simulink library "LIB_AirVolumeProcessing"  (R2018b)
settings: Solver=VariableStepAuto  StartTime=0.0  StopTime=10.0  RelTol=1e-3
undefined symbols (not defined in the file or in its folder): eRespiratorStates, QAirDeadZoneThd
libraries: simulink x9
settings Model: Creator=BRAUL  LastModifiedBy=VITIE

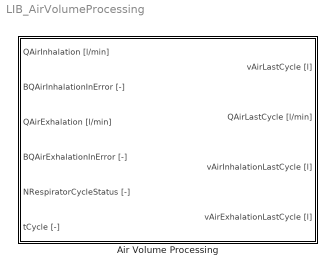
== system LIB_AirVolumeProcessing ==
  Air Volume Processing : Subsystem
      settings: AttributesFormatString=%<ReferenceBlock>

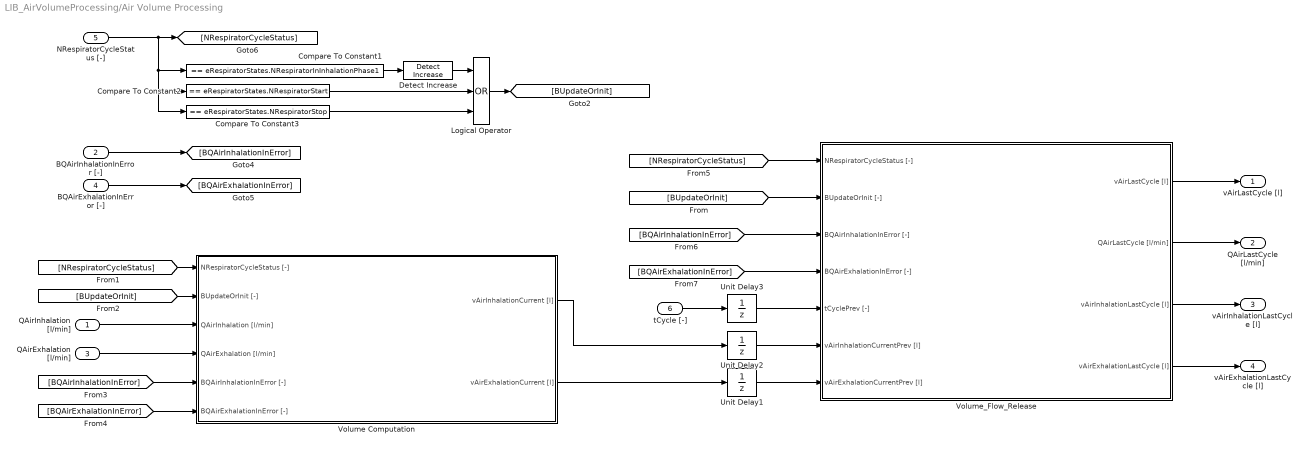
== system LIB_AirVolumeProcessing/Air Volume Processing ==
  QAirInhalation [l/min] : Inport
  BQAirInhalationInError [-] : Inport  Port=2
  QAirExhalation [l/min] : Inport  Port=3
  BQAirExhalationInError [-] : Inport  Port=4
  NRespiratorCycleStatus [-] : Inport  Port=5
  tCycle [-] : Inport  Port=6
  Compare To Constant1 : simulink/Logic and Bit Operations/Compare To Constant  relop===  const=eRespiratorStates.NRespiratorInInhalationPhase1  OutDataTypeStr=boolean
  Compare To Constant2 : simulink/Logic and Bit Operations/Compare To Constant  relop===  const=eRespiratorStates.NRespiratorStart  OutDataTypeStr=boolean
  Compare To Constant3 : simulink/Logic and Bit Operations/Compare To Constant  relop===  const=eRespiratorStates.NRespiratorStop  OutDataTypeStr=boolean
  Detect Increase : simulink/Logic and Bit Operations/Detect Increase  vinit=0.0  OutDataTypeStr=boolean
  Logical Operator : Logic  Operator=OR  Inputs=3  AllPortsSameDT=off  OutDataTypeStr=boolean
  Unit Delay1 : UnitDelay  SampleTime=-1
      settings: AttributesFormatString=%<InitialCondition>
  Unit Delay2 : UnitDelay  SampleTime=-1
      settings: AttributesFormatString=%<InitialCondition>
  Unit Delay3 : UnitDelay  SampleTime=-1
      settings: AttributesFormatString=%<InitialCondition>
  Volume Computation : Subsystem
  "Volume_Flow_Release " : Subsystem
  vAirLastCycle [l] : Outport
  QAirLastCycle [l/min] : Outport  Port=2
  vAirInhalationLastCycle [l] : Outport  Port=3
  vAirExhalationLastCycle [l] : Outport  Port=4
  wires:
  "Volume_Flow_Release "/3(vAirInhalationLastCycle [l]) -> vAirInhalationLastCycle [l]/1
  "Volume_Flow_Release "/4(vAirExhalationLastCycle [l]) -> vAirExhalationLastCycle [l]/1
  [BUpdateOrInit] -> "Volume_Flow_Release "/2(BUpdateOrInit [-])
  Compare To Constant3/1 -> Logical Operator/3
  Compare To Constant2/1 -> Logical Operator/2
  "Volume_Flow_Release "/1(vAirLastCycle [l]) -> vAirLastCycle [l]/1
  "Volume_Flow_Release "/2(QAirLastCycle [l/min]) -> QAirLastCycle [l/min]/1
  tCycle [-]/1 -> Unit Delay3/1
  Unit Delay3/1 -> "Volume_Flow_Release "/5(tCyclePrev [-])
  [BQAirInhalationInError] -> "Volume_Flow_Release "/3(BQAirInhalationInError [-])
  [BQAirExhalationInError] -> "Volume_Flow_Release "/4(BQAirExhalationInError [-])
  Volume Computation/1(vAirInhalationCurrent [l]) -> Unit Delay2/1
  Volume Computation/2(vAirExhalationCurrent [l]) -> Unit Delay1/1
  [BQAirExhalationInError] -> Volume Computation/6(BQAirExhalationInError [-])
  [BQAirInhalationInError] -> Volume Computation/5(BQAirInhalationInError [-])
  QAirExhalation [l/min]/1 -> Volume Computation/4(QAirExhalation [l/min])
  QAirInhalation [l/min]/1 -> Volume Computation/3(QAirInhalation [l/min])
  [NRespiratorCycleStatus] -> Volume Computation/1(NRespiratorCycleStatus [-])
  [BUpdateOrInit] -> Volume Computation/2(BUpdateOrInit [-])
  BQAirExhalationInError [-]/1 -> [BQAirExhalationInError]
  BQAirInhalationInError [-]/1 -> [BQAirInhalationInError]
  Unit Delay1/1 -> "Volume_Flow_Release "/7(vAirExhalationCurrentPrev [l])
  Unit Delay2/1 -> "Volume_Flow_Release "/6(vAirInhalationCurrentPrev [l])
  NRespiratorCycleStatus [-]/1 -> [NRespiratorCycleStatus], Compare To Constant3/1, Compare To Constant2/1, Compare To Constant1/1
  Compare To Constant1/1 -> Detect Increase/1
  Detect Increase/1 -> Logical Operator/1
  Logical Operator/1 -> [BUpdateOrInit]
  [NRespiratorCycleStatus] -> "Volume_Flow_Release "/1(NRespiratorCycleStatus [-])

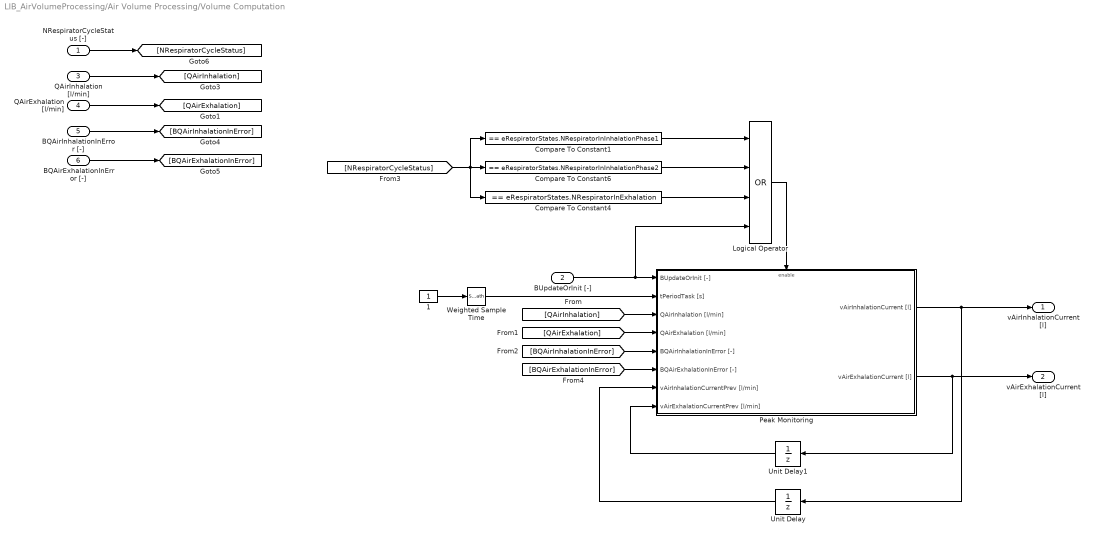
== system LIB_AirVolumeProcessing/Air Volume Processing/Volume Computation ==
  NRespiratorCycleStatus [-] : Inport
  BUpdateOrInit [-] : Inport  Port=2
  QAirInhalation [l/min] : Inport  Port=3
  QAirExhalation [l/min] : Inport  Port=4
  BQAirInhalationInError [-] : Inport  Port=5
  BQAirExhalationInError [-] : Inport  Port=6
  1 : Constant  OutDataTypeStr=single
  Compare To Constant1 : simulink/Logic and Bit Operations/Compare To Constant  relop===  const=eRespiratorStates.NRespiratorInInhalationPhase1  OutDataTypeStr=boolean
  Compare To Constant4 : simulink/Logic and Bit Operations/Compare To Constant  relop===  const=eRespiratorStates.NRespiratorInExhalation  OutDataTypeStr=boolean
  Compare To Constant6 : simulink/Logic and Bit Operations/Compare To Constant  relop===  const=eRespiratorStates.NRespiratorInInhalationPhase2  OutDataTypeStr=boolean
  Logical Operator : Logic  Operator=OR  Inputs=4  AllPortsSameDT=off  OutDataTypeStr=boolean
  Peak Monitoring : Subsystem
  Unit Delay : UnitDelay  SampleTime=-1
      settings: AttributesFormatString=%<InitialCondition>
  Unit Delay1 : UnitDelay  SampleTime=-1
      settings: AttributesFormatString=%<InitialCondition>
  Weighted Sample Time : SampleTimeMath  TsampMathOp=Ts Only  OutDataTypeStr=Inherit: Inherit via back propagation
  vAirInhalationCurrent [l] : Outport
  vAirExhalationCurrent [l] : Outport  Port=2
  wires:
  Compare To Constant4/1 -> Logical Operator/3
  Compare To Constant6/1 -> Logical Operator/2
  Compare To Constant1/1 -> Logical Operator/1
  [BQAirExhalationInError] -> Peak Monitoring/6(BQAirExhalationInError [-])
  [BQAirInhalationInError] -> Peak Monitoring/5(BQAirInhalationInError [-])
  [QAirExhalation] -> Peak Monitoring/4(QAirExhalation [l/min])
  [QAirInhalation] -> Peak Monitoring/3(QAirInhalation [l/min])
  Logical Operator/1 -> Peak Monitoring/Enable
  BQAirExhalationInError [-]/1 -> [BQAirExhalationInError]
  BQAirInhalationInError [-]/1 -> [BQAirInhalationInError]
  QAirExhalation [l/min]/1 -> [QAirExhalation]
  QAirInhalation [l/min]/1 -> [QAirInhalation]
  Weighted Sample Time/1 -> Peak Monitoring/2(tPeriodTask [s])
  1/1 -> Weighted Sample Time/1
  Unit Delay/1 -> Peak Monitoring/7(vAirInhalationCurrentPrev [l/min])
  Unit Delay1/1 -> Peak Monitoring/8(vAirExhalationCurrentPrev [l/min])
  Peak Monitoring/1(vAirInhalationCurrent [l]) -> Unit Delay/1, vAirInhalationCurrent [l]/1
  Peak Monitoring/2(vAirExhalationCurrent [l]) -> Unit Delay1/1, vAirExhalationCurrent [l]/1
  NRespiratorCycleStatus [-]/1 -> [NRespiratorCycleStatus]
  [NRespiratorCycleStatus] -> Compare To Constant6/1, Compare To Constant4/1, Compare To Constant1/1
  BUpdateOrInit [-]/1 -> Peak Monitoring/1(BUpdateOrInit [-]), Logical Operator/4

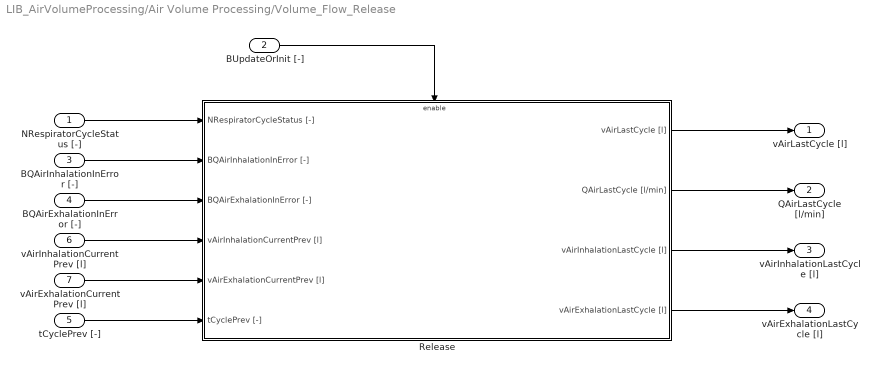
== system LIB_AirVolumeProcessing/Air Volume Processing/Volume_Flow_Release  ==
  NRespiratorCycleStatus [-] : Inport
  BUpdateOrInit [-] : Inport  Port=2
  BQAirInhalationInError [-] : Inport  Port=3
  BQAirExhalationInError [-] : Inport  Port=4
  tCyclePrev [-] : Inport  Port=5
  vAirInhalationCurrentPrev [l] : Inport  Port=6
  vAirExhalationCurrentPrev [l] : Inport  Port=7
  Release : Subsystem
  vAirLastCycle [l] : Outport
  QAirLastCycle [l/min] : Outport  Port=2
  vAirInhalationLastCycle [l] : Outport  Port=3
  vAirExhalationLastCycle [l] : Outport  Port=4
  wires:
  NRespiratorCycleStatus [-]/1 -> Release/1(NRespiratorCycleStatus [-])
  BUpdateOrInit [-]/1 -> Release/Enable
  Release/1(vAirLastCycle [l]) -> vAirLastCycle [l]/1
  Release/2(QAirLastCycle [l/min]) -> QAirLastCycle [l/min]/1
  vAirExhalationCurrentPrev [l]/1 -> Release/5(vAirExhalationCurrentPrev [l])
  vAirInhalationCurrentPrev [l]/1 -> Release/4(vAirInhalationCurrentPrev [l])
  BQAirExhalationInError [-]/1 -> Release/3(BQAirExhalationInError [-])
  BQAirInhalationInError [-]/1 -> Release/2(BQAirInhalationInError [-])
  tCyclePrev [-]/1 -> Release/6(tCyclePrev [-])
  Release/3(vAirInhalationLastCycle [l]) -> vAirInhalationLastCycle [l]/1
  Release/4(vAirExhalationLastCycle [l]) -> vAirExhalationLastCycle [l]/1

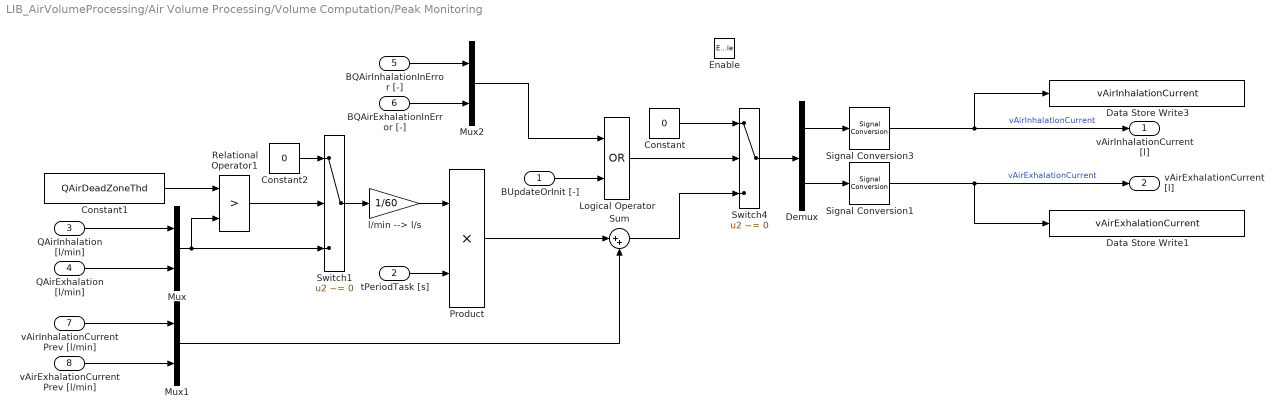
== system LIB_AirVolumeProcessing/Air Volume Processing/Volume Computation/Peak Monitoring ==
  BUpdateOrInit [-] : Inport
  tPeriodTask [s] : Inport  Port=2
  QAirInhalation [l/min] : Inport  Port=3
  QAirExhalation [l/min] : Inport  Port=4
  BQAirInhalationInError [-] : Inport  Port=5
  BQAirExhalationInError [-] : Inport  Port=6
  vAirInhalationCurrentPrev [l/min] : Inport  Port=7
  vAirExhalationCurrentPrev [l/min] : Inport  Port=8
  Enable : EnablePort
  Constant : Constant  Value=0  OutDataTypeStr=single
  Constant1 : Constant  Value=QAirDeadZoneThd
  Constant2 : Constant  Value=0  OutDataTypeStr=single
  Data Store Write1 : DataStoreWrite  DataStoreName=vAirExhalationCurrent
  Data Store Write3 : DataStoreWrite  DataStoreName=vAirInhalationCurrent
  Demux : Demux  Outputs=2
  Logical Operator : Logic  Operator=OR  AllPortsSameDT=off  OutDataTypeStr=boolean
  Mux : Mux  Inputs=2
  Mux1 : Mux  Inputs=2
  Mux2 : Mux  Inputs=2
  Product : Product
  Relational Operator1 : RelationalOperator  Operator=>  OutDataTypeStr=boolean  RndMeth=Simplest
  Signal Conversion1 : SignalConversion  OverrideOpt=off
  Signal Conversion3 : SignalConversion  OverrideOpt=off
  Sum : Sum  Inputs=|++
  Switch1 : Switch  Criteria=u2 ~= 0
      settings: AttributesFormatString=%<Criteria>
  Switch4 : Switch  Criteria=u2 ~= 0
      settings: AttributesFormatString=%<Criteria>
  l/min --> l/s : Gain  Gain=1/60
  vAirInhalationCurrent [l] : Outport
  vAirExhalationCurrent [l] : Outport  Port=2
  wires:
  Constant2/1 -> Switch1/1
  Relational Operator1/1 -> Switch1/2
  Switch1/1 -> l/min --> l/s/1
  Constant1/1 -> Relational Operator1/1
  Mux1/1 -> Sum/2
  Product/1 -> Sum/1
  BQAirInhalationInError [-]/1 -> Mux2/1
  BQAirExhalationInError [-]/1 -> Mux2/2
  Mux2/1 -> Logical Operator/1
  BUpdateOrInit [-]/1 -> Logical Operator/2
  Logical Operator/1 -> Switch4/2
  vAirInhalationCurrentPrev [l/min]/1 -> Mux1/1
  vAirExhalationCurrentPrev [l/min]/1 -> Mux1/2
  Demux/2 -> Signal Conversion1/1
  Signal Conversion1/1 -> vAirExhalationCurrent [l]/1, Data Store Write1/1  "vAirExhalationCurrent"
  Demux/1 -> Signal Conversion3/1
  Signal Conversion3/1 -> Data Store Write3/1, vAirInhalationCurrent [l]/1  "vAirInhalationCurrent"
  Switch4/1 -> Demux/1
  l/min --> l/s/1 -> Product/1
  QAirExhalation [l/min]/1 -> Mux/2
  Mux/1 -> Switch1/3, Relational Operator1/2
  QAirInhalation [l/min]/1 -> Mux/1
  tPeriodTask [s]/1 -> Product/2
  Constant/1 -> Switch4/1
  Sum/1 -> Switch4/3

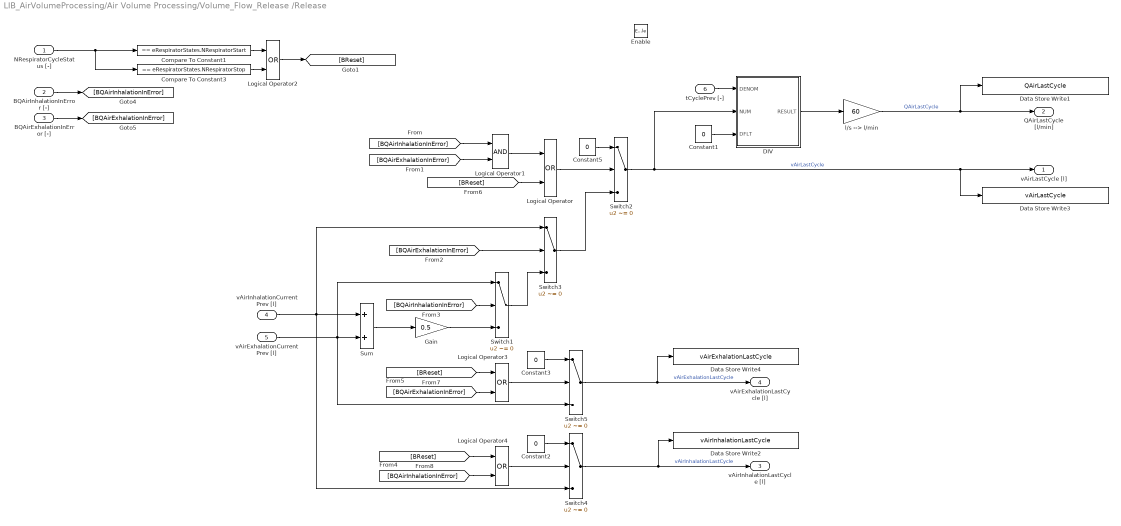
== system LIB_AirVolumeProcessing/Air Volume Processing/Volume_Flow_Release /Release ==
  NRespiratorCycleStatus [-] : Inport
  BQAirInhalationInError [-] : Inport  Port=2
  BQAirExhalationInError [-] : Inport  Port=3
  vAirInhalationCurrentPrev [l] : Inport  Port=4
  vAirExhalationCurrentPrev [l] : Inport  Port=5
  tCyclePrev [-] : Inport  Port=6
  Enable : EnablePort
  Compare To Constant1 : simulink/Logic and Bit Operations/Compare To Constant  relop===  const=eRespiratorStates.NRespiratorStart  OutDataTypeStr=boolean
  Compare To Constant3 : simulink/Logic and Bit Operations/Compare To Constant  relop===  const=eRespiratorStates.NRespiratorStop  OutDataTypeStr=boolean
  Constant{1..3,5} (4 alike) : Constant  Value=0  OutDataTypeStr=single
  DIV : Subsystem  mask(DIV){}
      mask help: This block executes a division with protection for division by 0.
      mask Display: disp('DIV')
  Data Store Write1 : DataStoreWrite  DataStoreName=QAirLastCycle
  Data Store Write2 : DataStoreWrite  DataStoreName=vAirInhalationLastCycle
  Data Store Write3 : DataStoreWrite  DataStoreName=vAirLastCycle
  Data Store Write4 : DataStoreWrite  DataStoreName=vAirExhalationLastCycle
  Gain : Gain  Gain=0.5
  Logical Operator{,2..4} (4 alike) : Logic  Operator=OR  AllPortsSameDT=off  OutDataTypeStr=boolean
  Logical Operator1 : Logic  AllPortsSameDT=off  OutDataTypeStr=boolean
  Sum : Sum
  Switch{1..5} (5 alike) : Switch  Criteria=u2 ~= 0
      settings: AttributesFormatString=%<Criteria>
  l/s --> l/min : Gain  Gain=60
  vAirLastCycle [l] : Outport
  QAirLastCycle [l/min] : Outport  Port=2
  vAirInhalationLastCycle [l] : Outport  Port=3
  vAirExhalationLastCycle [l] : Outport  Port=4
  wires:
  [BReset] -> Logical Operator4/1
  [BQAirInhalationInError] -> Logical Operator4/2
  Logical Operator4/1 -> Switch4/2
  [BReset] -> Logical Operator3/1
  [BQAirExhalationInError] -> Logical Operator3/2
  Logical Operator3/1 -> Switch5/2
  [BReset] -> Logical Operator/2
  Logical Operator2/1 -> [BReset]
  Compare To Constant3/1 -> Logical Operator2/2
  Compare To Constant1/1 -> Logical Operator2/1
  Switch4/1 -> Data Store Write2/1, vAirInhalationLastCycle [l]/1  "vAirInhalationLastCycle"
  Switch5/1 -> Data Store Write4/1, vAirExhalationLastCycle [l]/1  "vAirExhalationLastCycle"
  Constant3/1 -> Switch5/1
  Constant2/1 -> Switch4/1
  Switch2/1 -> DIV/2(NUM), vAirLastCycle [l]/1, Data Store Write3/1  "vAirLastCycle"
  l/s --> l/min/1 -> Data Store Write1/1, QAirLastCycle [l/min]/1  "QAirLastCycle"
  Constant1/1 -> DIV/3(DFLT)
  tCyclePrev [-]/1 -> DIV/1(DENOM)
  DIV/1(RESULT) -> l/s --> l/min/1
  Switch3/1 -> Switch2/3
  Switch1/1 -> Switch3/3
  [BQAirExhalationInError] -> Switch3/2
  [BQAirInhalationInError] -> Switch1/2
  vAirExhalationCurrentPrev [l]/1 -> Sum/2, Switch1/1, Switch5/3
  vAirInhalationCurrentPrev [l]/1 -> Sum/1, Switch3/1, Switch4/3
  Gain/1 -> Switch1/3
  Sum/1 -> Gain/1
  Logical Operator1/1 -> Logical Operator/1
  [BQAirExhalationInError] -> Logical Operator1/2
  [BQAirInhalationInError] -> Logical Operator1/1
  BQAirExhalationInError [-]/1 -> [BQAirExhalationInError]
  BQAirInhalationInError [-]/1 -> [BQAirInhalationInError]
  NRespiratorCycleStatus [-]/1 -> Compare To Constant3/1, Compare To Constant1/1
  Constant5/1 -> Switch2/1
  Logical Operator/1 -> Switch2/2

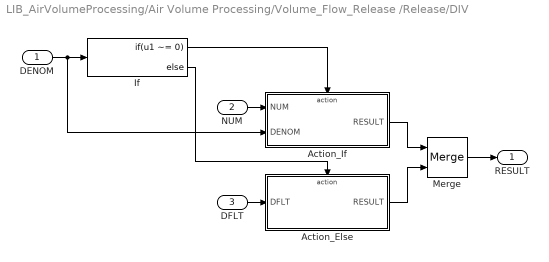
== system LIB_AirVolumeProcessing/Air Volume Processing/Volume_Flow_Release /Release/DIV ==
  DENOM : Inport
  NUM : Inport  Port=2
  DFLT : Inport  Port=3
  Action_Else : Subsystem  TreatAsAtomicUnit=on
  Action_If : Subsystem  TreatAsAtomicUnit=on
  If : If  IfExpression=u1 ~= 0
  Merge : Merge
  RESULT : Outport
  wires:
  Merge/1 -> RESULT/1
  Action_Else/1(RESULT) -> Merge/2
  Action_If/1(RESULT) -> Merge/1
  If/2 -> Action_Else/Action
  DFLT/1 -> Action_Else/1(DFLT)
  DENOM/1 -> If/1, Action_If/2(DENOM)
  NUM/1 -> Action_If/1(NUM)
  If/1 -> Action_If/Action

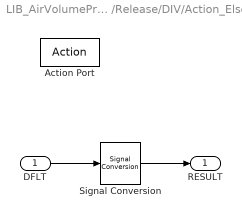
== system LIB_AirVolumeProcessing/Air Volume Processing/Volume_Flow_Release /Release/DIV/Action_Else ==
  DFLT : Inport
  Action Port : ActionPort
  Signal Conversion : SignalConversion  OverrideOpt=off
  RESULT : Outport
  wires:
  Signal Conversion/1 -> RESULT/1
  DFLT/1 -> Signal Conversion/1

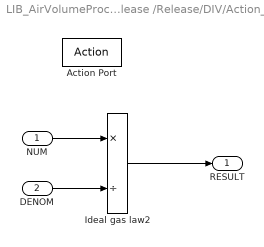
== system LIB_AirVolumeProcessing/Air Volume Processing/Volume_Flow_Release /Release/DIV/Action_If ==
  NUM : Inport
  DENOM : Inport  Port=2
  Action Port : ActionPort
  Ideal gas law2 : Product  Inputs=*/
  RESULT : Outport
  wires:
  DENOM/1 -> Ideal gas law2/2
  Ideal gas law2/1 -> RESULT/1
  NUM/1 -> Ideal gas law2/1
